simulink model "kde"  (R2022b)
settings: Solver=VariableStepAuto  StartTime=0.0  StopTime=orbit_E.T  RelTol=1e-9
values from neighbouring files (symbols this model uses):
  A0 = [1 0 0; 0 1 0; 0 0 1]    [test_script.m]
  earth_horizon = struct('dvst', 3*0.2 ,'accuracy', deg2rad(0.2))    [test_script.m]
  gyro = struct('c', 15e-3, 'ARW', 0.15, 'sigma_b', deg2rad(0.3) / 3600,                'freq', 262, 'accuracy', 2.4e-9)    [test_script.m]
  H0 = sqrt((-29615e-9)^2+(-1728e-9)^2+(5186e-9)^2)    [test_script.m]
  I = [Ix; Iy; Iz]    [test_script.m]
  Ir = 0.005    [test_script.m]
  K_d = 40 * Iz * 0.3 * orbit_E.n    [test_script.m]
  K_p = Iz * (20 * orbit_E.n)^2    [test_script.m]
  m_t = 5.9722e24    (= 5.9722e+24)    [test_script.m]
  Mr = 0    [test_script.m]
  orbit_E = struct('mu', astroConstants(13), 'a', astroConstants(23) + 2000,                    'e', 0.1, 'inc', deg2rad(10), 'G', astroConstants(1),                    'theta0', 0, 'R', astroConstants(23))    [test_script.m]
  orbit_S = struct('mu', astroConstants(4), 'a', astroConstants(2), 'e', 0.0167,                    'epsilon', deg2rad(23.45), 'G', astroConstants(1),                    'theta0', 0  )    [test_script.m]
  r = pos-pos_CG    [test_script.m]
  solarPanel = struct( 'r', r, 'P', radiation/(3e8),                      'rho_d', .1, 'rho_s', [.5, .5, .5, .5, .5 .5, .1, .1, .1, .1],                      'area', [.06 .06 .04 .06 .06 .04 .12 .12 .12 .12])    [test_script.m]
  sun_sensor = struct('dvst', 3*0.2 ,'accuracy', deg2rad(0.2))    [test_script.m]
  w0 = [0; 0; orbit_E.n]    [test_script.m]
  wr0 = 0    [test_script.m]
undefined symbols (not defined in the file or in its folder): a_e, e, e_e, inc, T_e, theta0, w_e
libraries: matrix_library x5, vrlib x3, simulink_extras x1, dspinverses x1
(part 2 of 2)

== system kde/Subsystem/Actuator/state observer/Subsystem1/Subsystem3 ==
  B : Inport
  A : Inport  Port=2
  C : Inport  Port=3
  Gain : Gain  Gain=-1
  MATLAB Function : MATLAB Function  TreatAsAtomicUnit=on
  MatrixMultiply : Product  Multiplication=Matrix(*)
  MatrixMultiply1 : Product  Multiplication=Matrix(*)
  L : Outport
  wires:
  C/1 -> MATLAB Function/3(C)
  B/1 -> MatrixMultiply/1, MATLAB Function/1(B)
  MatrixMultiply/1 -> MatrixMultiply1/2
  MATLAB Function/1(P) -> MatrixMultiply1/1
  MatrixMultiply1/1 -> Gain/1
  Gain/1 -> L/1  "L"
  A/1 -> MATLAB Function/2(A)
  MATLAB Function/2(R) -> MatrixMultiply/2

== system kde/Subsystem/Attitude Determination/Subsystem2/Subsystem/true anomaly ==
  Constant : Constant  Value=orbit_E.theta0
  Constant1 : Constant  Value=orbit_E.n
  Constant10 : Constant  Value=3/2
  Constant8 : Constant
  Constant9 : Constant
  Cos : Trigonometry  Operator=cos
  Integrator : Integrator  InitialConditionSource=external
  Power : Math  Operator=pow
  Product1 : Product
  Product2 : Product
  Product3 : Product  Inputs=*/
  Square : Math  Operator=square
  Square1 : Math  Operator=square
  Sum : Sum  Inputs=|++
  Sum1 : Sum  Inputs=|-+
  eccentricity : Constant  Value=orbit_E.e
  theta : Outport
  wires:
  eccentricity/1 -> Square1/1, Product1/2
  Sum1/1 -> Power/1
  Product3/1 -> Integrator/1  "theta_dot"
  Constant9/1 -> Sum1/2
  Constant8/1 -> Sum/2
  Square1/1 -> Sum1/1
  Square/1 -> Product2/1
  Sum/1 -> Square/1
  Product2/1 -> Product3/1
  Cos/1 -> Product1/1
  Power/1 -> Product3/2
  Constant10/1 -> Power/2
  Integrator/1 -> theta/1, Cos/1  "theta"
  Constant/1 -> Integrator/2
  Product1/1 -> Sum/1
  Constant1/1 -> Product2/2

== system kde/Subsystem/Attitude Determination/Subsystem2/sun distance magnitude/true anomaly ==
  Constant : Constant  Value=orbit_S.theta0
  Constant1 : Constant  Value=orbit_S.n
  Constant10 : Constant  Value=3/2
  Constant8 : Constant
  Constant9 : Constant
  Cos : Trigonometry  Operator=cos
  Integrator : Integrator  InitialConditionSource=external
  Power : Math  Operator=pow
  Product1 : Product
  Product2 : Product
  Product3 : Product  Inputs=*/
  Square : Math  Operator=square
  Square1 : Math  Operator=square
  Sum : Sum  Inputs=|++
  Sum1 : Sum  Inputs=|-+
  eccentricity : Constant  Value=orbit_S.e
  theta : Outport
  n_sun : Outport  Port=2
  wires:
  Sum/1 -> Square/1
  Product1/1 -> Sum/1
  Integrator/1 -> theta/1, Cos/1  "theta"
  Cos/1 -> Product1/1
  Square/1 -> Product2/1
  Constant8/1 -> Sum/2
  Square1/1 -> Sum1/1
  eccentricity/1 -> Square1/1, Product1/2
  Constant10/1 -> Power/2
  Sum1/1 -> Power/1
  Constant9/1 -> Sum1/2
  Power/1 -> Product3/2
  Product3/1 -> Integrator/1  "theta_dot"
  Product2/1 -> Product3/1
  Constant/1 -> Integrator/2
  Constant1/1 -> n_sun/1, Product2/2

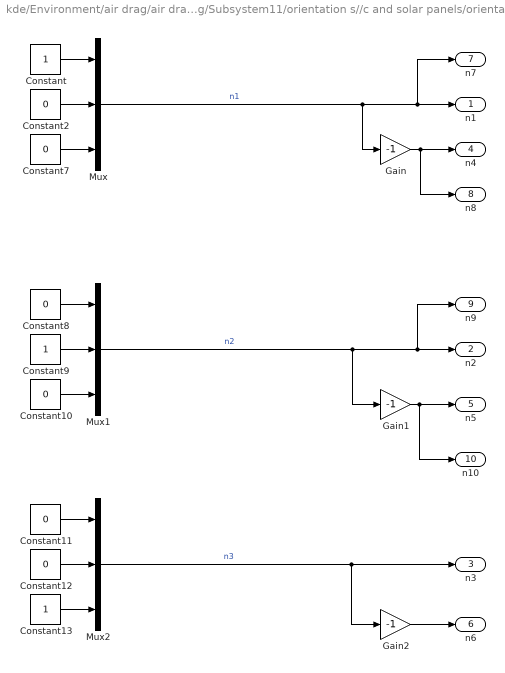
== system kde/Environment/air drag/air drag/Subsystem11/orientation s//c and solar panels/orientation s//c and solar panels in B ==
  Constant : Constant
  Constant{2,7..8,10..12} (6 alike) : Constant  Value=0
  Constant13 : Constant
  Constant9 : Constant
  Gain : Gain  Gain=-1
  Gain1 : Gain  Gain=-1
  Gain2 : Gain  Gain=-1
  Mux : Mux  Inputs=3
  Mux1 : Mux  Inputs=3
  Mux2 : Mux  Inputs=3
  n1 : Outport
  n2 : Outport  Port=2
  n3 : Outport  Port=3
  n4 : Outport  Port=4
  n5 : Outport  Port=5
  n6 : Outport  Port=6
  n7 : Outport  Port=7
  n8 : Outport  Port=8
  n9 : Outport  Port=9
  n10 : Outport  Port=10
  wires:
  Mux1/1 -> Gain1/1, n9/1, n2/1  "n2"
  Mux2/1 -> n3/1, Gain2/1  "n3"
  Constant7/1 -> Mux/3
  Constant9/1 -> Mux1/2
  Gain1/1 -> n10/1, n5/1
  Gain/1 -> n8/1, n4/1
  Mux/1 -> Gain/1, n7/1, n1/1  "n1"
  Constant11/1 -> Mux2/1
  Constant12/1 -> Mux2/2
  Gain2/1 -> n6/1
  Constant13/1 -> Mux2/3
  Constant10/1 -> Mux1/3
  Constant2/1 -> Mux/2
  Constant/1 -> Mux/1
  Constant8/1 -> Mux1/1

== matlab function kde/Environment/air drag/air drag/Subsystem11/MATLAB Function ==
  data: v_rel_1 input; y output; N input; v_rel input
function y = fcn(v_rel_1, N, v_rel)

F = zeros(3, 10);

for i = 1:10

    if dot(N(:, i), v_rel_1) < 0
        F(:, i) = zeros(3, 1);
    else
        F(:, i) = -0.5 * rho_air * c_d * norm(v_rel)^2;% * dot(N(:, i), v_rel_1) * area(i);% .* v_rel_1;
    end

end

y = sum(F');

== matlab function kde/Subsystem/Actuator/state observer/MATLAB Function ==
  data: I input; A output; C output; n input; B output
function [A, C, B] = fcn(I, n)

Ix = I(1);
Iy = I(2);
Iz = I(3);

Kx = (Iz - Iy) / Ix;
Ky = (Iz - Ix) / Iy;

A = [    0,     1,          0,      0,      0, 0;
     -Kx*n^2,   0,          0,    (1-Kx)*n, 0, 0;
         0,     0,          0,      1,      0, 0;
         0,   (Ky-1)*n,  -Ky*n^2,   0,      0, 0;
         0,     0,          0,      0,      0, 1;
         0,     0,          0,      0,      0, 0];

B = [ 0,    0,    0;
     1/Ix,  0,    0;
      0,    0,    0;
      0,   1/Iy,  0;
      0,    0,    0;
      0,    0,   1/Iz];

C = [0, 1, -n, 0, 0, 0;
     0, n,  0, 1, 0, 0;
     0, 0,  0, 0, 0, 1];

end

== matlab function kde/Environment/air drag/air drag/MATLAB Function ==
  data: w input; y output; r input
function y = fcn(w, r)

u = zeros(10, 3);

for i = 1:10
    u(i, :) = cross(w, r(:, i));
end

y = sum(u);

== matlab function kde/Subsystem/Attitude Determination/MATLAB Function ==
  data: B input; U output; M output; V output
function [U, M, V] = fcn(B)

[U, S, V] = svd(B);
M = diag([1, 1, det(U)*det(V)]);

end

== matlab function kde/Environment/srp disturbance/Subsystem/MATLAB Function1 ==
  data: F input; pos input; T_SRP output; cond input
function T_SRP = fcn(F, pos, cond)

T = zeros(length(cond),3);

for i = 1:length(cond)
    if cond(i) > 0
        T(i,:) = cross(pos(:,i), F(:,i));
    end
end

T_sum = sum(T);

T_SRP = T_sum;

== matlab function kde/Subsystem/Actuator/state observer/Subsystem1/Subsystem3/MATLAB Function ==
  data: B input; P output; A input; C input; R output
function [P, R] = fcn(B, A, C)

% Algebraic riccati equation

Q = C'*C;
P = zeros(6, 6);

coder.extrinsic('idare');

% [P, K, L_eig] 
P = idare(A, B, Q, [], [], [], []);
R = eye(3);

% P is such that L = -PB*inv(R)
% K = state feedback gains
% L_eig closed loops eigenvalues
